simulink model "task_4_controller"  (R2024a)
settings: Solver=VariableStepAuto  StartTime=0.0  StopTime=1000  RelTol=1e-3
values from neighbouring files (symbols this model uses):
  A = sys.A    [task4.m]    (also in task4_old.m = zeros(6, 6))
  B = sys.B    [task4.m]    (also in task4_old.m = zeros(6,2))
  C = sys.C    [task4.m]    (also in task4_old.m = zeros(2,6))
  K = (P*C')*R2    [task4.m]    (also in task4_old.m; task6.m = (P*C')/R2)
  L = (1\Q2)*B'*S    [task4.m]    (also in task4_old.m; task6.m = inv(Q2)*(Bnom')*S)
  Lr = inv(M*inv((B*L -A))*B)    [task4.m]    (also in task4_old.m; task6.m)
undefined symbols (not defined in the file or in its folder): linear_params
settings Model: PacingRate=22  Creator=geopap-4  LastModifiedBy=geopap-4

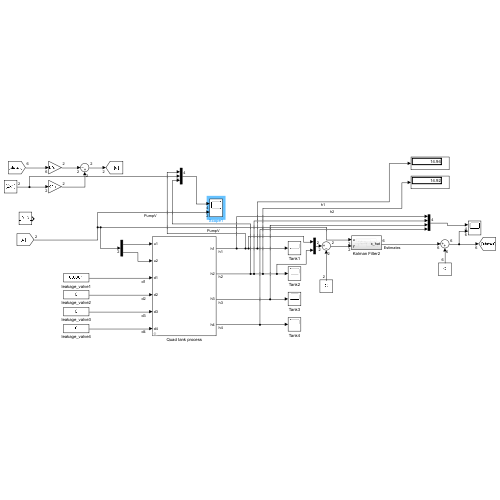
[thumbnail: Simulink's stored preview of the top-level diagram]
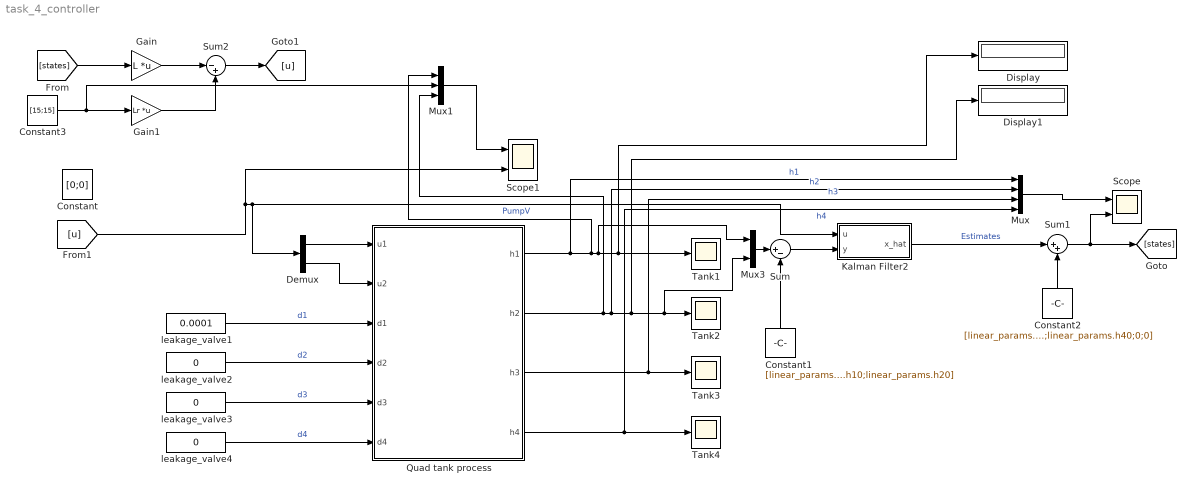
== system task_4_controller ==
  Constant : Constant  Value=[0;0]
  Constant1 : Constant  Value=[linear_params.h10;linear_params.h20]
  Constant2 : Constant  Value=[linear_params.h10;linear_params.h20;linear_params.h30;linear_params.h40;0;0]
  Constant3 : Constant  Value=[15;15]
  Demux : Demux  Outputs=2
  Display : Display
  Display1 : Display
  Gain : Gain  Gain=L  Multiplication=Matrix(K*u)
  Gain1 : Gain  Gain=Lr  Multiplication=Matrix(K*u)
  Kalman Filter2 : Subsystem
  Mux : Mux
  Mux1 : Mux  Inputs=3
  Mux3 : Mux  Inputs=2
  Quad tank process : Subsystem  mask{hmax=20, A1=28, ao1=0.071, h10=0, A2=32, ao2=0.057, h20=0, A3=28, ao3=0.071, h30=0, A4=32, ao4=0.057, h40=0, k1=3.33, k2=3.35, gamma1=0.7, gamma2=0.6}
      mask prompts: hmax "Tank height (cm)"; A1 "Tank area (cm^2)"; ao1 "Opening area (cm^2)"; h10 "Initial level (cm)"; A2 "Tank area (cm^2)"; ao2 "Opening area (cm^2)"; h20 "Initial level (cm)"; A3 "Tank area (cm^2)"; ao3 "Opening area (cm^2)"; h30 "Initial level (cm)"; A4 "Tank area (cm^2)"; ao4 "Opening area (cm^2)"; h40 "Initial level (cm)"; k1 "Pump1 gain (cm^3/V/s)"; k2 "Pump2 gain (cm^3/V/s)"; gamma1 "Split valve gamma 1"; gamma2 "Split valve gamma 2"
      mask help: Double tank process parameters
      mask DialogControl Container3 Prompt: General parameters
      mask DialogControl ParameterGroupVar Prompt: Tank 1
      mask DialogControl ParameterGroupVar_copy_copy_copy Prompt: Tank 2
      mask DialogControl ParameterGroupVar_copy_copy Prompt: Tank 3
      mask DialogControl ParameterGroupVar_copy Prompt: Tank 4
      mask DialogControl Container4 Prompt: Pump parameters
  Scope : Scope  NumInputPorts=2
  Scope1 : Scope  NumInputPorts=2
  Sum : Sum  Inputs=|+-
  Sum1 : Sum  Inputs=|++
  Sum2 : Sum  Inputs=|-+
  Tank{1..4} (4 alike) : Scope
  leakage_valve1 : Constant  Value=0.0001
  leakage_valve2 : Constant  Value=0
  leakage_valve3 : Constant  Value=0
  leakage_valve4 : Constant  Value=0
  wires:
  leakage_valve2/1 -> Quad tank process/4(d2)  "d2"
  leakage_valve3/1 -> Quad tank process/5(d3)  "d3"
  Quad tank process/2(h2) -> Mux1/3, Mux/2, Display1/1, Mux3/2, Tank2/1  "h2"
  leakage_valve1/1 -> Quad tank process/3(d1)  "d1"
  leakage_valve4/1 -> Quad tank process/6(d4)  "d4"
  Quad tank process/4(h4) -> Mux/4, Tank4/1  "h4"
  Quad tank process/3(h3) -> Mux/3, Tank3/1  "h3"
  Quad tank process/1(h1) -> Mux/1, Mux1/1, Mux3/1, Display/1, Tank1/1  "h1"
  Demux/1 -> Quad tank process/1(u1)
  Demux/2 -> Quad tank process/2(u2)
  [u] -> Scope1/2, Demux/1, Kalman Filter2/1(u)  "PumpV"
  Kalman Filter2/1(x_hat) -> Sum1/1  "Estimates"
  Sum/1 -> Kalman Filter2/2(y)
  Constant1/1 -> Sum/2
  Mux3/1 -> Sum/1
  Sum1/1 -> Scope/2, [states]
  Constant2/1 -> Sum1/2
  [states] -> Gain/1
  Gain/1 -> Sum2/1
  Gain1/1 -> Sum2/2
  Constant3/1 -> Mux1/2, Gain1/1
  Sum2/1 -> [u]
  Mux1/1 -> Scope1/1
  Mux/1 -> Scope/1

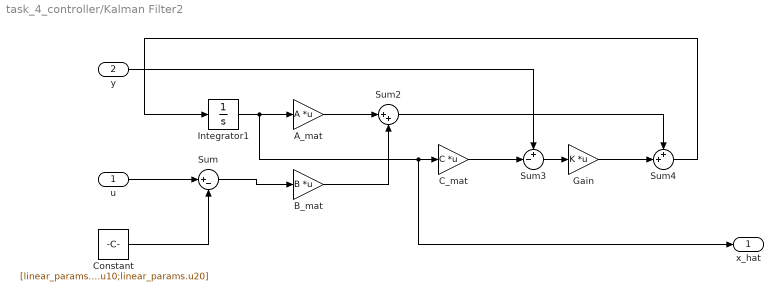
== system task_4_controller/Kalman Filter2 ==
  u : Inport
  y : Inport  Port=2
  A_mat : Gain  Gain=A  Multiplication=Matrix(K*u)
  B_mat : Gain  Gain=B  Multiplication=Matrix(K*u)
  C_mat : Gain  Gain=C  Multiplication=Matrix(K*u)
  Constant : Constant  Value=[linear_params.u10;linear_params.u20]
  Gain : Gain  Gain=K  Multiplication=Matrix(K*u)
  Integrator1 : Integrator
  Sum : Sum  Inputs=|+-
  Sum2 : Sum  Inputs=|++
  Sum3 : Sum  Inputs=+-|
  Sum4 : Sum  Inputs=++|
  x_hat : Outport
  wires:
  y/1 -> Sum3/1
  Gain/1 -> Sum4/2
  A_mat/1 -> Sum2/1
  Integrator1/1 -> x_hat/1, C_mat/1, A_mat/1
  Sum3/1 -> Gain/1
  Sum2/1 -> Sum4/1
  B_mat/1 -> Sum2/2
  Sum4/1 -> Integrator1/1
  C_mat/1 -> Sum3/2
  u/1 -> Sum/1
  Sum/1 -> B_mat/1
  Constant/1 -> Sum/2

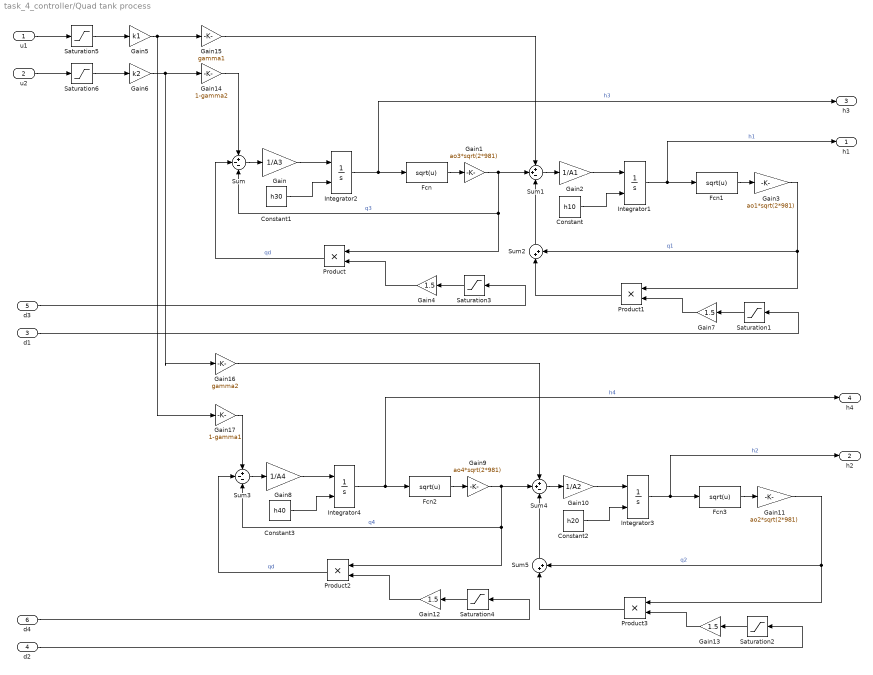
== system task_4_controller/Quad tank process ==
  u1 : Inport
  u2 : Inport  Port=2
  d1 : Inport  Port=3
  d2 : Inport  Port=4
  d3 : Inport  Port=5
  d4 : Inport  Port=6
  Constant : Constant  Value=h10
  Constant1 : Constant  Value=h30
  Constant2 : Constant  Value=h20
  Constant3 : Constant  Value=h40
  Fcn{,1..3} (4 alike) : Fcn  Expr=sqrt(u)
  Gain : Gain  Gain=1/A3
  Gain1 : Gain  Gain=ao3*sqrt(2*981)
  Gain10 : Gain  Gain=1/A2
  Gain11 : Gain  Gain=ao2*sqrt(2*981)
  Gain{4,7,12..13} (4 alike) : Gain  Gain=1.5
  Gain14 : Gain  Gain=1-gamma2
  Gain15 : Gain  Gain=gamma1
  Gain16 : Gain  Gain=gamma2
  Gain17 : Gain  Gain=1-gamma1
  Gain2 : Gain  Gain=1/A1
  Gain3 : Gain  Gain=ao1*sqrt(2*981)
  Gain5 : Gain  Gain=k1
  Gain6 : Gain  Gain=k2
  Gain8 : Gain  Gain=1/A4
  Gain9 : Gain  Gain=ao4*sqrt(2*981)
  Integrator{1..4} (4 alike) : Integrator  InitialConditionSource=external  LimitOutput=on  UpperSaturationLimit=hmax  LowerSaturationLimit=0
  Product{,1..3} (4 alike) : Product  RndMeth=Zero
  Saturation{1..4} (4 alike) : Saturate  UpperLimit=1  LowerLimit=0
  Saturation5 : Saturate  UpperLimit=10  LowerLimit=0
  Saturation6 : Saturate  UpperLimit=10  LowerLimit=0
  Sum : Sum  Inputs=+--
  Sum1 : Sum  Inputs=++-
  Sum2 : Sum  Inputs=|++
  Sum3 : Sum  Inputs=+--
  Sum4 : Sum  Inputs=++-
  Sum5 : Sum  Inputs=|++
  h1 : Outport  VectorParamsAs1DForOutWhenUnconnected=off
  h2 : Outport  Port=2  VectorParamsAs1DForOutWhenUnconnected=off
  h3 : Outport  Port=3  VectorParamsAs1DForOutWhenUnconnected=off
  h4 : Outport  Port=4  VectorParamsAs1DForOutWhenUnconnected=off
  wires:
  Sum/1 -> Gain/1
  Gain/1 -> Integrator2/1
  Fcn/1 -> Gain1/1
  Gain1/1 -> Product/1, Sum/3, Sum1/2  "q3"
  Sum1/1 -> Gain2/1
  Gain2/1 -> Integrator1/1
  Fcn1/1 -> Gain3/1
  Integrator2/1 -> h3/1, Fcn/1  "h3"
  Product/1 -> Sum/2  "qd"
  d3/1 -> Saturation3/1
  Integrator1/1 -> h1/1, Fcn1/1  "h1"
  Saturation3/1 -> Gain4/1
  Gain4/1 -> Product/2
  u1/1 -> Saturation5/1
  Constant/1 -> Integrator1/2
  Constant1/1 -> Integrator2/2
  u2/1 -> Saturation6/1
  Gain5/1 -> Gain17/1, Gain15/1
  Sum2/1 -> Sum1/3
  Gain3/1 -> Product1/1, Sum2/2  "q1"
  Gain7/1 -> Product1/2
  Saturation1/1 -> Gain7/1
  d1/1 -> Saturation1/1
  Product1/1 -> Sum2/1
  Product3/1 -> Sum5/1
  d2/1 -> Saturation2/1
  Saturation2/1 -> Gain13/1
  Gain13/1 -> Product3/2
  Gain11/1 -> Sum5/2, Product3/1  "q2"
  Sum5/1 -> Sum4/3
  Constant3/1 -> Integrator4/2
  Constant2/1 -> Integrator3/2
  Gain12/1 -> Product2/2
  Saturation4/1 -> Gain12/1
  Integrator3/1 -> Fcn3/1, h2/1  "h2"
  d4/1 -> Saturation4/1
  Product2/1 -> Sum3/2  "qd"
  Integrator4/1 -> h4/1, Fcn2/1  "h4"
  Fcn3/1 -> Gain11/1
  Gain10/1 -> Integrator3/1
  Sum4/1 -> Gain10/1
  Gain9/1 -> Sum4/2, Sum3/3, Product2/1  "q4"
  Fcn2/1 -> Gain9/1
  Gain8/1 -> Integrator4/1
  Sum3/1 -> Gain8/1
  Gain14/1 -> Sum/1
  Gain15/1 -> Sum1/1
  Gain6/1 -> Gain16/1, Gain14/1
  Gain16/1 -> Sum4/1
  Gain17/1 -> Sum3/1
  Saturation5/1 -> Gain5/1
  Saturation6/1 -> Gain6/1
